simulink subsystem "ManualTest"  (R2024a)
settings: Solver=VariableStepAuto  StartTime=0.0  StopTime=10.0  RelTol=1e-3
libraries: px4lib x3
settings Model: Creator=gurt1  LastModifiedBy=gurt1

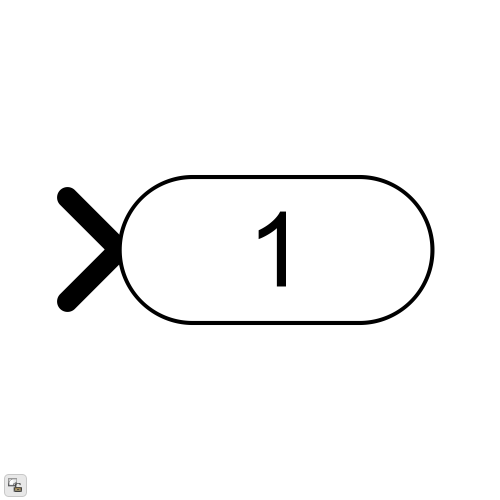
[thumbnail: Simulink's stored preview of the top-level diagram]
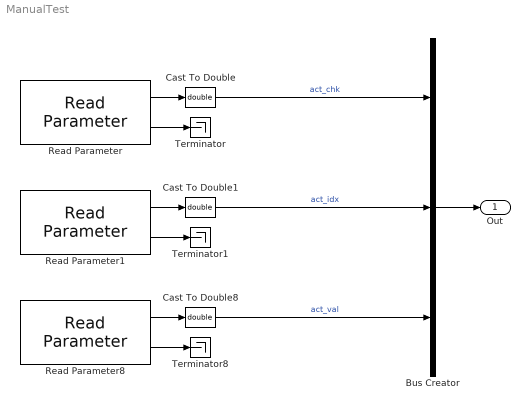
== system ManualTest ==
  Bus Creator : BusCreator  Inputs=3
  Cast To Double : DataTypeConversion  OutDataTypeStr=double  SaturateOnIntegerOverflow=off  RndMeth=Floor
  Cast To Double1 : DataTypeConversion  OutDataTypeStr=double  SaturateOnIntegerOverflow=off  RndMeth=Floor
  Cast To Double8 : DataTypeConversion  OutDataTypeStr=double  SaturateOnIntegerOverflow=off  RndMeth=Floor
  Read Parameter : px4lib/Read Parameter  ParameterName=MANUAL_ACT_CHK  DataType=FLOAT  SampleTime=-1
  Read Parameter1 : px4lib/Read Parameter  ParameterName=MANUAL_ACT_IDX  DataType=FLOAT  SampleTime=-1
  Read Parameter8 : px4lib/Read Parameter  ParameterName=MANUAL_ACT_VAL  DataType=FLOAT  SampleTime=-1
  Terminator : Terminator
  Terminator1 : Terminator
  Terminator8 : Terminator
  Out : Outport
  wires:
  Read Parameter/2 -> Terminator/1
  Read Parameter/1 -> Cast To Double/1
  Cast To Double/1 -> Bus Creator/1  "act_chk"
  Read Parameter1/1 -> Cast To Double1/1
  Read Parameter1/2 -> Terminator1/1
  Cast To Double1/1 -> Bus Creator/2  "act_idx"
  Cast To Double8/1 -> Bus Creator/3  "act_val"
  Read Parameter8/1 -> Cast To Double8/1
  Read Parameter8/2 -> Terminator8/1
  Bus Creator/1 -> Out/1
